simulink model "V4_Modell_Wagen_Validierung_Matlab_ver_R2022a"  (R2022a)
settings: Solver=ode3  StartTime=0.0  StopTime=Zeit(end)  FixedStep=0.001  RelTol=1e-3
values from neighbouring files (symbols this model uses):
  k_M = C_Phi    (= 42.43)    [V4_Parameter_Parameter_komplett_te.m]    (also in V4_Parameter_Wagen_Te.m = -0.04243; V4_Parameter_komplett.m = -0.04243)
  r_ZR = 0.021    [V4_Parameter_Parameter_komplett_te.m]    (also in V4_Parameter_Wagen_Te.m; V4_Parameter_komplett.m)
settings Model: Creator=JSCHB  LastModifiedBy=Patrick
settings ModelReferenceCC: EnableRefExpFcnMdlSchedulingChecks=off
settings RTWCC: Description=Generic Real-Time Target

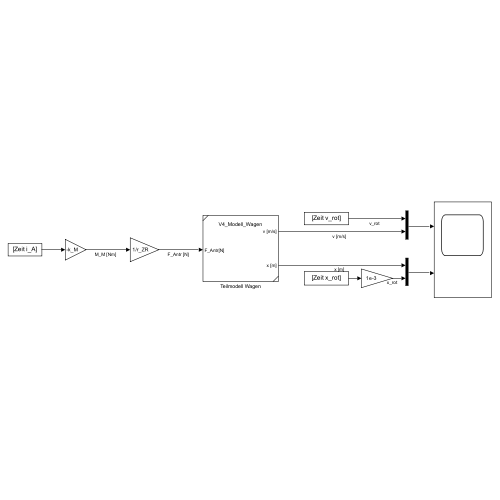
[thumbnail: Simulink's stored preview of the top-level diagram]
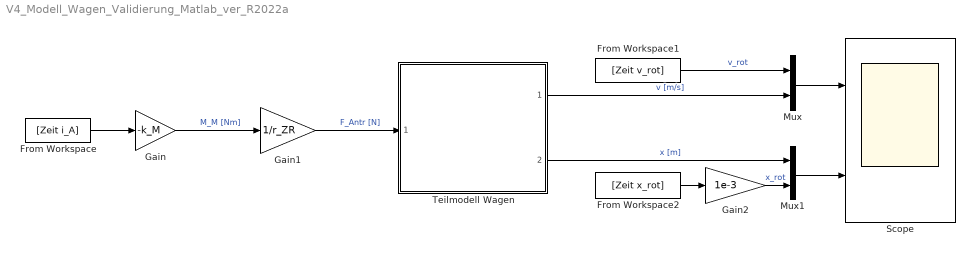
== system V4_Modell_Wagen_Validierung_Matlab_ver_R2022a ==
  From Workspace : FromWorkspace  VariableName=[Zeit i_A]
  From Workspace1 : FromWorkspace  VariableName=[Zeit v_rot]
  From Workspace2 : FromWorkspace  VariableName=[Zeit x_rot]
  Gain : Gain  Gain=-k_M
  Gain1 : Gain  Gain=1/r_ZR
  Gain2 : Gain  Gain=1e-3
  Mux : Mux  Inputs=2
  Mux1 : Mux  Inputs=2
  Scope : Scope  NumInputPorts=2
  Teilmodell Wagen : Subsystem  ReferencedSubsystem=V4_Modell_Wagen
  wires:
  Gain/1 -> Gain1/1  "M_M [Nm]"
  Gain1/1 -> Teilmodell Wagen/1  "F_Antr [N]"
  From Workspace/1 -> Gain/1
  Teilmodell Wagen/1 -> Mux/2  "v [m/s]"
  Teilmodell Wagen/2 -> Mux1/1  "x [m]"
  From Workspace1/1 -> Mux/1  "v_rot"
  From Workspace2/1 -> Gain2/1
  Gain2/1 -> Mux1/2  "x_rot"
  Mux/1 -> Scope/1
  Mux1/1 -> Scope/2
